simulink model "s_tanks_3_CL"  (R2016b)
settings: Solver=FixedStepAuto  StartTime=0.0  StopTime=400  FixedStep=Ts  RelTol=1e-3  EnableMultiTasking=on
values from neighbouring files (symbols this model uses):
  gamma = Ai2 / ( Ai1 + Ai2 )    [d_tanks_3.m]
  step_time = 100    [Identificacion_T3.m]    (also in Identificacion_T3_S2.m)
  Ts = 0.01    [Identificacion_T3.m]    (also in Identificacion_T3_S2.m)
undefined symbols (not defined in the file or in its folder): Ao1, Ao2, At1, At2, g, Kp, VMAX_AMP
libraries: simulink x1, mpclib x1
settings Model: ExtModeTrigDuration=60000  Creator=MLevis  LastModifiedBy=cristobal
settings SolverCC: PositivePriorityOrder=on
settings DataIOCC: LimitDataPoints=on  SaveFormat=Array  SignalLoggingSaveFormat=ModelDataLogs
settings OptimizationCC: ExpressionDepthLimit=2147483647  InitFltsAndDblsToZero=on  LifeSpan=inf
settings DebuggingCC: SaveWithParameterizedLinksMsg=none  UnderspecifiedInitializationDetection=Classic  MergeDetectMultiDrivingBlocksExec=none  SolverPrmCheckMsg=warning  FcnCallInpInsideContextMsg=warning  StateNameClashWarn=warning  SFUnexpectedBacktrackingDiag=warning  SFNoUnconditionalDefaultTransitionDiag=warning  SFExecutionAtInitializationDiag=none
settings HardwareCC: ProdBitPerPointer=32  ProdBitPerSizeT=32  ProdBitPerPtrDiffT=32  ProdLargestAtomicFloat=None  ProdIntDivRoundTo=Undefined  ProdEndianess=Unspecified  ProdWordSize=32  ProdHWDeviceType=32-bit Generic
settings ModelReferenceCC: PropagateSignalLabelsOutOfModel=off
settings RTWCC: SystemTargetFile=quarc_windows.tlc  TemplateMakefile=quarc_default_tmf  Description=QuaRC Win32 Target
settings STFCustomTargetCC: TargetFcnLib=ansi_tfl_tmw.mat  TargetPreCompLibLocation=C:\PROGRA~3\QUARC\lib\2012b\windows\release  GeneratePreprocessorConditionals=Disable all  CPPClassGenCompliant=on  SystemTargetFile=quarc_windows.tlc
settings GRTTargetCC: TargetFcnLib=ansi_tfl_tmw.mat  TargetPreCompLibLocation=C:\PROGRA~3\QUARC\lib\2012b\windows\release  TargetLangStandard=C89/C90 (ANSI)  ParMdlRefBuildCompliant=off  CompOptLevelCompliant=off  ConcurrentExecutionCompliant=off  GeneratePreprocessorConditionals=Disable all  CombineOutputUpdateFcns=off  MatFileLogging=off  GRTInterface=on  UseToolchainInfoCompliant=off  ExtMode=on  ExtModeMexFile=quarc_comm
settings ConfigComp: CovMetricSettings=dw  CovHtmlReporting=on  CovSaveCumulativeToWorkspaceVar=on  CovSaveSingleToWorkspaceVar=on  CovExternalEMLEnable=off

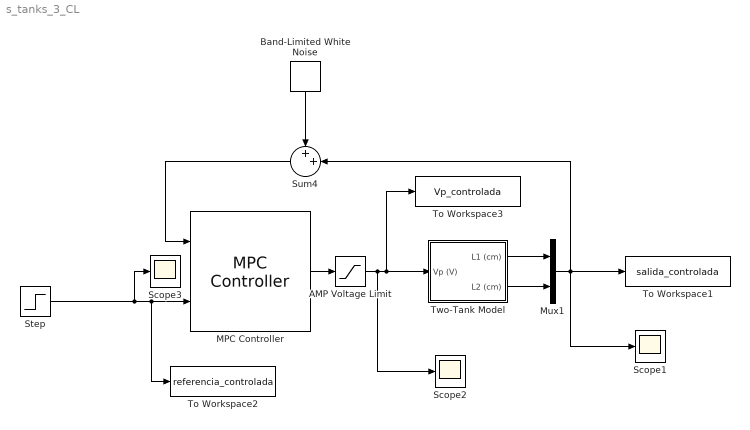
== system s_tanks_3_CL ==
  AMP Voltage Limit : Saturate  UpperLimit=VMAX_AMP  LowerLimit=0
  Band-Limited White Noise : simulink/Sources/Band-Limited White Noise  Cov=N_power  Ts=Ts  seed=[23341]
  MPC Controller : mpclib/MPC Controller  SCDEnableBlockLinearizationSpecification=on  mpcobj=mpcobj  is_multiple=0  enable_value=0  return_u0=off  ref_from_ws=off  ref_signal_name=[]  ref_preview=off  md_from_ws=off  md_signal_name=[]  md_preview=off  from_project=off  project_file=MPCtask.mat  md_inport=off  mv_inport=off  cost_outport=off  return_sequence=off  return_qpstatus=off  return_state=off  state_inport=off  lims_inport=off  ywt_inport=off  is_designfromscratch=0  uwt_inport=off  duwt_inport=off  rhoeps_inport=off  uref_inport=off  n_ts=0.01  n_mv=1  n_md=0  n_ud=0  n_mo=2  n_uo=0  BlockDataType=double  SampleTimeInherited=off  switch_inport=off
  Mux1 : Mux  Inputs=2
  Scope1 : Scope
  Scope2 : Scope
  Scope3 : Scope
  Step : Step  Time=step_time  Before=[15 15]  After=step  SampleTime=0
  Sum4 : Sum  Inputs=++|  SaturateOnIntegerOverflow=on  InputSameDT=on  OutDataTypeStr=Inherit: Same as first input
  To Workspace1 : ToWorkspace  VariableName=salida_controlada  SaveFormat=Timeseries  SampleTime=-1
  To Workspace2 : ToWorkspace  VariableName=referencia_controlada  SaveFormat=Timeseries  SampleTime=-1
  To Workspace3 : ToWorkspace  VariableName=Vp_controlada  SaveFormat=Timeseries  SampleTime=-1
  Two-Tank Model : Subsystem
  wires:
  Mux1/1 -> Sum4/2, Scope1/1, To Workspace1/1
  Step/1 -> Scope3/1, To Workspace2/1, MPC Controller/2
  MPC Controller/1 -> AMP Voltage Limit/1
  Two-Tank Model/1(L1 (cm)) -> Mux1/1
  Two-Tank Model/2(L2 (cm)) -> Mux1/2
  AMP Voltage Limit/1 -> Scope2/1, To Workspace3/1, Two-Tank Model/1(Vp (V))
  Sum4/1 -> MPC Controller/1
  Band-Limited White Noise/1 -> Sum4/1

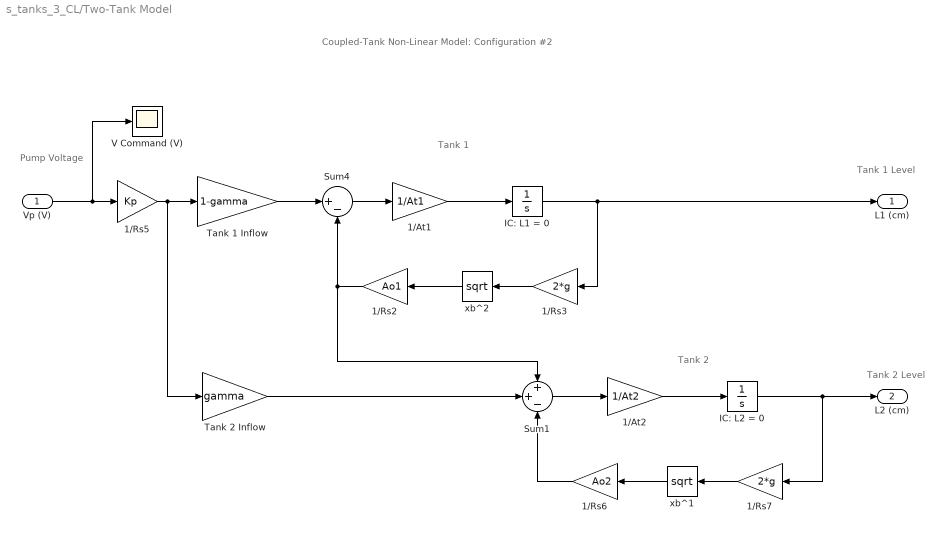
== system s_tanks_3_CL/Two-Tank Model ==
  note: Pump
      | Voltage
  note: Tank 1 Level
  note: Tank 2 Level
  note: Tank 2
  note: Tank 1
  note: Coupled-Tank Non-Linear Model:
      | Configuration #2
  Vp (V) : Inport
  1/At1 : Gain  Gain=1/At1  SaturateOnIntegerOverflow=on  OutDataTypeStr=Inherit: Same as input  ParamDataTypeStr=Inherit: Same as input
  1/At2 : Gain  Gain=1/At2  SaturateOnIntegerOverflow=on  OutDataTypeStr=Inherit: Same as input  ParamDataTypeStr=Inherit: Same as input
  1/Rs2 : Gain  Gain=Ao1  SaturateOnIntegerOverflow=on  OutDataTypeStr=Inherit: Same as input  ParamDataTypeStr=Inherit: Same as input
  1/Rs3 : Gain  Gain=2*g  SaturateOnIntegerOverflow=on  OutDataTypeStr=Inherit: Same as input  ParamDataTypeStr=Inherit: Same as input
  1/Rs5 : Gain  Gain=Kp  SaturateOnIntegerOverflow=on  OutDataTypeStr=Inherit: Same as input  ParamDataTypeStr=Inherit: Same as input
  1/Rs6 : Gain  Gain=Ao2  SaturateOnIntegerOverflow=on  OutDataTypeStr=Inherit: Same as input  ParamDataTypeStr=Inherit: Same as input
  1/Rs7 : Gain  Gain=2*g  SaturateOnIntegerOverflow=on  OutDataTypeStr=Inherit: Same as input  ParamDataTypeStr=Inherit: Same as input
  IC: L1 = 0 : Integrator
  IC: L2 = 0 : Integrator
  Sum1 : Sum  Inputs=++-  SaturateOnIntegerOverflow=on  InputSameDT=on  OutDataTypeStr=Inherit: Same as first input
  Sum4 : Sum  Inputs=|+-  SaturateOnIntegerOverflow=on  InputSameDT=on  OutDataTypeStr=Inherit: Same as first input
  Tank 1 Inflow : Gain  Gain=1-gamma
  Tank 2 Inflow : Gain  Gain=gamma
  V Command (V) : Scope
  xb^1 : Math  Operator=sqrt  SaturateOnIntegerOverflow=on
  xb^2 : Math  Operator=sqrt  SaturateOnIntegerOverflow=on
  L1 (cm) : Outport  InitialOutput=0
  L2 (cm) : Outport  Port=2  InitialOutput=0
  wires:
  1/Rs7/1 -> xb^1/1
  xb^1/1 -> 1/Rs6/1
  IC: L2 = 0/1 -> L2 (cm)/1, 1/Rs7/1
  1/At2/1 -> IC: L2 = 0/1
  Sum1/1 -> 1/At2/1
  1/Rs3/1 -> xb^2/1
  xb^2/1 -> 1/Rs2/1
  1/Rs2/1 -> Sum4/2, Sum1/1
  IC: L1 = 0/1 -> L1 (cm)/1, 1/Rs3/1
  1/At1/1 -> IC: L1 = 0/1
  Sum4/1 -> 1/At1/1
  Vp (V)/1 -> 1/Rs5/1, V Command (V)/1
  1/Rs6/1 -> Sum1/3
  1/Rs5/1 -> Tank 1 Inflow/1, Tank 2 Inflow/1
  Tank 1 Inflow/1 -> Sum4/1
  Tank 2 Inflow/1 -> Sum1/2
